simulink model "chap17_02_97_mdl"  (R2013b)
settings: Solver=FixedStepDiscrete  StartTime=0.0  StopTime=10.0  FixedStep=0.1  RelTol=1e-3
settings Model: Creator=Administrator  LastModifiedBy=sunzx.fnst
settings OptimizationCC: OptimizeModelRefInitCode=on  LifeSpan=1
settings RTWCC: SystemTargetFile=ert.tlc  GenCodeOnly=on  TemplateMakefile=ert_default_tmf  Description=Embedded Coder  GenerateReport=on  ProcessScript=ert_make_rtw_hook  IncludeHyperlinkInReport=on  LaunchReport=on
settings CodeAppCC: IgnoreCustomStorageClasses=off
settings ERTTargetCC: CodeReplacementLibrary=ANSI_C  GenerateSampleERTMain=on  ERTCustomFileTemplate=example_file_process.tlc  EnableUserReplacementTypes=on

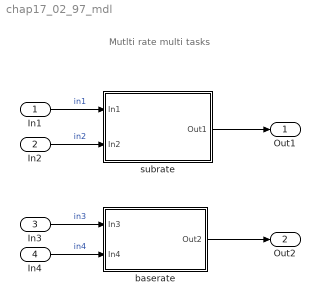
== system chap17_02_97_mdl ==
  note: Mutlti rate multi tasks
  In1 : Inport  OutDataTypeStr=FLOAT32
  In2 : Inport  Port=2  OutDataTypeStr=UINT16
  In3 : Inport  Port=3  OutDataTypeStr=FLOAT32
  In4 : Inport  Port=4  OutDataTypeStr=UINT16
  baserate : Subsystem  TreatAsAtomicUnit=on
      settings: RTWFcnNameOpts=Use subsystem name
  subrate : Subsystem  TreatAsAtomicUnit=on  SystemSampleTime=0.6
      settings: RTWFcnNameOpts=Use subsystem name
  Out1 : Outport  OutDataTypeStr=boolean
  Out2 : Outport  Port=2  OutDataTypeStr=boolean
  wires:
  In3/1 -> baserate/1(In3)  "in3"
  In4/1 -> baserate/2(In4)  "in4"
  baserate/1(Out2) -> Out2/1
  In1/1 -> subrate/1(In1)  "in1"
  In2/1 -> subrate/2(In2)  "in2"
  subrate/1(Out1) -> Out1/1

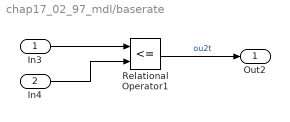
== system chap17_02_97_mdl/baserate ==
  In3 : Inport  OutDataTypeStr=FLOAT32
  In4 : Inport  Port=2  OutDataTypeStr=UINT16
  Relational Operator1 : RelationalOperator  Operator=<=  OutDataTypeStr=boolean
  Out2 : Outport  OutDataTypeStr=boolean
  wires:
  Relational Operator1/1 -> Out2/1  "ou2t"
  In3/1 -> Relational Operator1/1
  In4/1 -> Relational Operator1/2

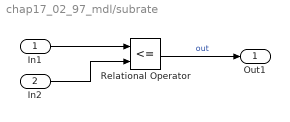
== system chap17_02_97_mdl/subrate ==
  In1 : Inport  OutDataTypeStr=FLOAT32
  In2 : Inport  Port=2  OutDataTypeStr=UINT16
  Relational Operator : RelationalOperator  Operator=<=  OutDataTypeStr=boolean
  Out1 : Outport
  wires:
  In2/1 -> Relational Operator/2
  In1/1 -> Relational Operator/1
  Relational Operator/1 -> Out1/1  "out"
